simulink model "decisionTask"  (R2012b)
settings: Solver=FixedStepDiscrete  StartTime=0.0  StopTime=10.0  FixedStep=0.001  RelTol=1e-3
undefined symbols (not defined in the file or in its folder): acquireMethods, autoplayMovementDuration, autoplayReactionTime, autoplayRotationDuration, autoplayRotationStart, centerOffset, clickPercentage, clickRefractoryPeriod, clickTargetColor, clickTargetHoverColor, coherences, crossSize, cuedText, cuedTextLength, cumulativeDwell, cursorColorClick, cursorColorClosed, cursorColorOpen, cursorColors, cursorDiameter, cursorNeuralColor, cursorNonneuralColor, delayOrder, delayPeriodGainScale, displayObject, doHeadSpeedFail, drawNumbersOnTargets, dwellRefractoryPeriod, errorAssistAxis, errorAssistR, errorAssistTheta, expRandBinSize, expRandMax, expRandMin, expRandMu, eyeMode, failOnLiftoff, failurePenalty, falseClickFails, fingerPositionTolerance, fixedSeqMode, freePlayMode, gain, gloveBias, gloveLPDenominator, gloveLPNumerator, gloveNonlinearCorrection, gloveXCorrection, gloveYCorrection, gracePeriod, gridEdges, gridSize, gridTilesEachDim, headSpeedCap, holdDuration, holdTime, initialInput, initialLockout, initialState, inputType ... (+118)
(part 2 of 2)

== matlab function decisionTask/decisionTaskSplit ==
  data: xkRaw input double size=[double(xkConstants.NUM_STATE_DIMENSIONS) 1]; xkMod input; behaviorPacket input Bus: behaviorPacketBus size=1; vizData input Bus: peripheralData; taskOutput output Bus: taskOutput; stateParameters input Bus: stateParams size=1; decisionParameters input Bus: taskParamsBus; clock input; xpcTET input; xkModBiasEst input; taskAgnosticXk input; xkAux input
function taskOutput  = decisionTaskSplit(xkRaw, xkMod, behaviorPacket, vizData,  ...
    stateParameters, decisionParameters, clock, xpcTET, xkModBiasEst, taskAgnosticXk, xkAux)
% removed from input: clickState, clickParameters,
% should I change the connectors in the model to match this change? - SNF
%#codegen
% This is the state-machine-like implementation of the cursor task.
% This, depending on paraemters, can do center-out-and-back
%
% October 31 2016: now has two state inputs, xkRaw (which gets fed back to
% the decoder), and xkMod. Generally should look at xkMod for task logic,
% but if the game needs to change a state element which ought to propogate
% into the decoder (for example re-seed the cursor), it should do this to
% both xkRaw and xkMod.

% decisionParameters is actually taskParamsBus, which is set by
% cursotTask_buildWorkspace.m

%% INITIALIZE TASK OUTPUT - SNF to SNF: don't fuck with this.
fileLoggerData.data = uint8(zeros(1,1400));
fileLoggerData.dataLen = uint16(0);
fileLoggerData.fileName = uint8(zeros(1,20));
fileLoggerData.send = false;

fileLoggerFormat.format = uint8(zeros(1,1400));
fileLoggerFormat.formatLen = uint16(0);
fileLoggerFormat.fileName = uint8(zeros(1,20));

fileLoggerFormatAndData.format = fileLoggerFormat;
fileLoggerFormatAndData.data = fileLoggerData;

%% whether or not to allow the cursor to be stopped (e.g. during click)
% allowStop = true;
% resetHMM = false;

taskOutput.flushFiles = false;
taskOutput.sendFormat = false;
taskOutput.taskDetails = fileLoggerFormat;
taskOutput.discrete = fileLoggerFormatAndData;
taskOutput.continuous = fileLoggerFormatAndData;
taskOutput.screen = fileLoggerFormatAndData;
taskOutput.sound = fileLoggerFormatAndData;
taskOutput.asynch = fileLoggerFormatAndData;
taskOutput.ttl = double(0);
taskOutput.xk = xkRaw;
taskOutput.inputType = decisionParameters.initialInput;
taskOutput.currentTarget = single(zeros([double(xkConstants.NUM_TARGET_DIMENSIONS) 1]));
taskOutput.state = uint16(CursorStates.STATE_INIT);
taskOutput.paused = false;
taskOutput.allowStop =  true; %allowStop;
taskOutput.resetHMM = false; %resetHMM;

%% TASK DETAILS PACKET: SNF done for DM, builds successfully
TASK_NAME = 'decision';
VERSION_ID = single(0.01); % Alpha - SF

taskOutput.taskDetails = packFileLoggerTaskDetails(TASK_NAME, VERSION_ID, ...
    'STATE_INIT', uint8(CursorStates.STATE_INIT), ...
    'STATE_PRE_TRIAL', uint8(CursorStates.STATE_PRE_TRIAL),...
    'STATE_NEW_TARGET', uint8(CursorStates.STATE_NEW_TARGET),...
    'STATE_MOVE', uint8(CursorStates.STATE_MOVE),...
    'STATE_ACQUIRE', uint8(CursorStates.STATE_ACQUIRE),...
    'STATE_SUCCESS', uint8(CursorStates.STATE_SUCCESS),...
    'STATE_FAIL', uint8(CursorStates.STATE_FAIL),...
    'STATE_CENTER_TARGET', uint8(CursorStates.STATE_CENTER_TARGET),...
    'STATE_END', uint8(CursorStates.STATE_END),...
    'STATE_RECENTER_DELAY', uint8(CursorStates.STATE_RECENTER_DELAY),...
    'STATE_FIXATE', uint8(CursorStates.STATE_FIXATE),... %SNF DM state
    'STATE_STIMULUS_ONSET', uint8(CursorStates.STATE_STIMULUS_ONSET),... %SNF DM state
    'STATE_INTERTRIAL',  uint8(CursorStates.STATE_INTERTRIAL),... %SNF DM state
    'INPUT_TYPE_HEAD_MOUSE', uint8(cursorConstants.INPUT_TYPE_HEAD_MOUSE),...
    'INPUT_TYPE_CURSOR_HEADSTILL', uint8(cursorConstants.INPUT_TYPE_CURSOR_HEADSTILL),...%SF changed this 4/12
    'INPUT_TYPE_NONE', uint8(cursorConstants.INPUT_TYPE_NONE),... %SF: probably need this?
    'OUTPUT_TYPE_CURSOR', uint8(cursorConstants.OUTPUT_TYPE_CURSOR)...
    );

%% TASK-RELATED CONSTANTS
NUM_DIMS =  uint8(cursorConstants.NUM_DIMENSIONS); %this is 5
headCursorPos = single( zeros(1,NUM_DIMS) ); % head position cursor
cursorAlpha2 = uint8(100); % set to 100 if you're not using it. This is in %.

INIT_LENGTH = uint16(100); %ms
% PRE_TRIAL_LENGTH = uint16(20); %ms
SCORE_LENGTH = uint16(4000); %ms
INIT_TIME = uint32(2000); %this one's used explicitly for keeping pauseTriggered
MAX_MOVE_TIME = uint32(10000);
% HEAD_CURSOR_COLOR = [0; 204; 102;];
% AUTOPLAY_COLOR = [255; 255; 255];
EYE_X_SCALAR = 1680;
EYE_Y_SCALAR = 1050;
%HEAD_SCALAR = 1080; %this is only for offline I think
%%% DM specific
GRID_SIZE = 15*15; 
ISOGREEN = [0 90 0];
ISORED   = [160 0 0];
COLORMAT = [ISORED; ISOGREEN];
% trialConds: always L/D and Red first. 
% idx 1: 2 = L/R, 1 = U/D
% idx 2: color of left or down targ (depending on col 1) 2 = red, 3 = green
% idx 3: color of right or up targ  (depending on col 1) 2 = red, 3 = green
% idx 4: number of red squares (out of 225)
% idx 5: which target is correct. 1 = left/up, 2 = right/down
%indices into stimulus conditions matrix:
TARG_AXIS_IDX = 1;
LEFT_DN_TARG_COLOR_IDX = 2; %subtract 1 to get index for target order. left/down always first
RIGHT_UP_TARG_COLOR_IDX = 3; %always the second entry
NUM_RED_SQ_IDX = 4;
TARGET_LOC_IDX = 5;
% specifies what the values for each column mean:
LEFT_RIGHT_AXIS_TARGS = 2;
UP_DOWN_AXIS_TARGS = 1;
TARGET_RED = 2; %minus 1 to get row in COLORMAT
TARGET_GREEN = 3;  %minus 1 to get row in COLORMAT
LEFT_DN_TARG_S = 1;
RIGHT_UP_TARG_S = 2;
LEFT_DN_TARG_IDX = 1;
RIGHT_UP_TARG_IDX = 2;
% indices for activeTargs mask: could be more clever 
% DOWN_IDX = 1; why use these when the targAxis works
% LEFT_IDX = 2; 
% UP_IDX = 3; 
% RIGHT_IDX = 4;
CENTER_IDX = 5; 
% colors for those: 
TARGET_WHITE = 1;
TARGET_BLACK = 0; 
MIN_STIM_TIME = 300; 
%% DEFINE PERSISTENTS
persistent state vizPacket;
persistent pauseTriggered;
persistent stateTimer;
persistent holdTimer;
%persistent cursorColors; %this is defined in the task now
persistent targetRadiusTrans % added SDS Feb 2017, this is the target radius in XYZ
persistent targetRadiusRot % added SDS Feb 2017, this is the target radius in rotation
persistent currentTarget;
persistent nextTarget;
persistent speedCode;
persistent wiaCode; %this needs to stay for reasons SNF doesn't know

%persistent currentTargetType nextTargetType;  % dwell or click
persistent trialNum %cycleNum cycleIndex;
persistent trialDelayLength;

persistent localAcquired localTotal localTotalTime localAcqTime;
%persistent localScore totalScore;
persistent acquireTime lastState;

persistent lockedParameters inputType outputType;

persistent lastSoundTime;
persistent lastSoundState;

%persistent initialeffectorCursorPos; % previousInput;

persistent totalTaskTime;
%persistent lastAcquireSuccess 
persistent previousTarget;
persistent filteredHeadSpeed;
persistent prevHeadPos;
persistent lastHeadSpeedFail;

 
%DM-specific:
% persistent gracePeriod; % this should go in the params file SNF TO SDS HELP PLZ
% persistent maxStimDur; % ditto. 
persistent stimConds; % This didn't make it into the param script
% persistent moveThresh; % ditto again. 
% persistent intertrialTime; %last one- in the params plz
persistent trialConds;
persistent fixDur;  % variable timed
persistent targDur; % variable timed
persistent stimulusCount; %trialNum might replace this? 
persistent successPoints;
%defining targets:
persistent targAxis;
persistent targColors; %numTargs x RGB 
persistent targLocs;   %numTargs x XY
persistent autoTarg; % 1 or 2 for L/D or R/U 
%defining stimulus:
persistent numRedSquares; 
persistent activeTargs; 
persistent maxFixateAttemptTime; 
persistent fixateAttemptTimer; 
persistent autoCursorPos; 
%% grab these off the bus: 

behaviorRequestClock = behaviorPacket.xpcRequestClock;
peripheralTimestamp = behaviorPacket.peripheralTimestamp(1:16);

%% INITIALIZE PERSISTENTS
if(isempty(state))
    state = uint16(CursorStates.STATE_INIT);
    lastState = state;
    currentTarget = single(zeros([double(xkConstants.NUM_TARGET_DIMENSIONS) 1]));
    nextTarget = single(zeros([double(xkConstants.NUM_TARGET_DIMENSIONS) 1]));
    
    speedCode = uint16(0); %FRW hacky instructed speed experiment
    wiaCode = uint16(0); %FRW hacky wia experiment
    vizPacket = initVizPacket;
    stateTimer = uint16(0);
    holdTimer = int16(0);
    pauseTriggered = true;
    
  %  cursorColors = double(zeros([3 3])); % there's a second cursor (column 2) allowed; now a third for eye cursor
    filteredHeadSpeed = single(0);
    prevHeadPos = single(zeros(2,1));
    
    %% buffer all the parameters off the bus
    lockedParameters = decisionParameters;
    stimConds = getStimMat(double(lockedParameters.coherences)); %this only happens once per run of the task.
    targetRadiusTrans = (double(lockedParameters.targetDiameter) / 2) +(double(lockedParameters.cursorDiameter) / 2);
    targetRadiusRot = double(lockedParameters.targetRotDiameter) / 2;
    
    inputType = lockedParameters.initialInput;
    trialNum = uint16(0);
  %  cycleNum = uint16(0);
  %  cycleIndex = uint16(1); % 1 so it's a valid idnex even when first used
    trialDelayLength = uint16(0);
    
    localTotal = uint16(0);
    localTotalTime = uint16(0);
    localAcquired = uint16(0);
    localAcqTime = uint16(0);
    acquireTime = stateTimer;
   % currentTargetType = uint16(cursorConstants.TARGET_TYPE_DWELL);
    nextTargetType = uint16(cursorConstants.TARGET_TYPE_DWELL);
    %SFstateBeforePreTrial = uint16(0);
    lastSoundTime = clock;
    lastSoundState = uint8(CursorStates.SOUND_STATE_IDLE);

    
    totalTaskTime = uint32(0);
    lastHeadSpeedFail = uint32(0);
    
 %   lastAcquireSuccess = false;
    previousTarget = currentTarget;
    % DM-specific: 
    fixDur = uint16(0); 
    targDur = uint16(0); 
    successPoints = uint16(0);
    stimulusCount = uint16(1); 
    %initialize stimulus conditions
    targAxis = uint16(LEFT_RIGHT_AXIS_TARGS);
    trialConds = uint16(zeros(1,5));
    targColors = uint16(zeros(2, 3)); 
    targColors(LEFT_DN_TARG_COLOR_IDX -1,:)  = uint16(ISORED); % if I see two red targets I know it's a problem
    targColors(RIGHT_UP_TARG_COLOR_IDX -1,:) = uint16(ISORED); % but we at least got here
    numRedSquares = uint16(GRID_SIZE); %if all red, again, we know we got here. 
    targLocs = single(zeros(2,2)); 
    targLocs(:, LEFT_DN_TARG_COLOR_IDX -1) = single([-1; -1]); %one target in the lower left, one in upper right. Col = targ
    targLocs(:, RIGHT_UP_TARG_COLOR_IDX -1) = single([1; 1]);
   % gracePeriod = uint16(200); %ms
    autoTarg = uint16(0); % no target
   % maxStimDur = uint16(0); 
   % moveThresh = uint16(200); %units of idk mate
   % intertrialTime = uint16(1000); %ms 
 %  activeTargs = logical(false(1,5)); 
   activeTargs = uint16(zeros(1,5)); 
   maxFixateAttemptTime = uint16(5000); %ms
   fixateAttemptTimer = uint16(0); 
   autoCursorPos =  double(zeros(5,1));
end

%% some more initialization
if(clock < INIT_TIME) %1 whole second
    pauseTriggered = true;
end
%% inits per loop: 
outputType = decisionParameters.outputType; % determines what graphics engine will render this task.
% We usually shouldn't write discrete data
writeDiscreteData = false; %only gets set to true in state_pre_trial once
writeContinuousData = true;

if(vizData.receive && (vizData.dataLen > 0 ))
    vizPacket = parseVizPacket(vizData.data);
end

% set the cursor and target color
% if uint16(inputType) == uint16(cursorConstants.INPUT_TYPE_HEAD_MOUSE)
%     cursorColors(1:end,1) = [0; 204; 102;]; %head position is always green
% elseif  uint16(inputType) == uint16(cursorConstants.INPUT_TYPE_AUTO_ACQUIRE)
%     cursorColors(1:end,1) = [255; 255; 255]; % BCI control
% end
targetColor = 'a'; % in other tasks, target still aqua
makeGridFlag = uint16(0);
% init target logic- transient 
translateOnTargetLD = false; 
translateOnTargetRU = false; 
%% some end effector maths
% which state elements do I look to for the cursor's position? SDS July 2016
xk2HorizontalPos = uint8( lockedParameters.xk2HorizontalPos );
xk2VerticalPos = uint8( lockedParameters.xk2VerticalPos );
xk2HorizontalVel = uint8( lockedParameters.xk2HorizontalVel );
xk2VerticalVel = uint8( lockedParameters.xk2VerticalVel );
xk2DepthPos = uint8( lockedParameters.xk2DepthPos );
xk2DepthVel = uint8( lockedParameters.xk2DepthVel );
xk2RotatePos = uint8( lockedParameters.xk2RotatePos );
xk2RotateVel = uint8( lockedParameters.xk2RotateVel );
xk2Rotate2Pos = uint8( lockedParameters.xk2Rotate2Pos );
xk2Rotate2Vel = uint8( lockedParameters.xk2Rotate2Vel );
TASK_DIMS = lockedParameters.numDisplayDims; % 2. only used for determining what kind of
% checking to use. We still need to have everything be NUM_DIMS (5) long or
% things won't compile.
canBePosInds = [xk2HorizontalPos,xk2VerticalPos,xk2DepthPos,xk2RotatePos,xk2Rotate2Pos];
canBeVelInds = [xk2HorizontalVel,xk2VerticalVel,xk2DepthVel,xk2RotateVel,xk2Rotate2Vel];
effectorPosInds = canBePosInds(1:NUM_DIMS);
effectorVelInds = canBeVelInds(1:NUM_DIMS);

%displayAuxCursor = false;
if uint16(inputType) == uint16(cursorConstants.INPUT_TYPE_HEAD_MOUSE)
    effectorPos = xkMod(effectorPosInds); %Head position is the main effector
    effectorVel = xkMod(effectorVelInds); %lol head vel not saved
    %auxEffectorPos = xkMod(effectorPosInds); %BCI is auxilary. 
    %auxEffectorPos = zeros(NUM_DIMS,1);    %Actually no, we don't care about BCI
    auxEffectorPos = effectorPos; %make this easy for SNF and PTB- always send head pos as cursor2
    %displayAuxCursor = true; %the head cursor *is* the cursor, so no aux
    %cursorColors(:,2) = AUTOPLAY_COLOR; %HEAD_CURSOR_COLOR; %SF doesn't want a green cursor in a red/green task
%elseif uint16(inputType) == uint16(cursorConstants.INPUT_TYPE_AUTO_ACQUIRE)
elseif uint16(inputType) == uint16(cursorConstants.INPUT_TYPE_CURSOR_HEADSTILL)
    effectorPos = xkMod(effectorPosInds); %BCI is the main effector
    effectorVel = xkMod(effectorVelInds);
    auxEffectorPos = xkAux(effectorPosInds); %head mouse is auxEffector
    %displayAuxCursor = true; %only show head cursor during fixation
    %cursorColors(:,2) = AUTOPLAY_COLOR; % BCI control
else %default to BCI and dgaf about head position
    effectorPos = xkMod(effectorPosInds);
    effectorVel = xkMod(effectorVelInds);
    auxEffectorPos = zeros(NUM_DIMS,1);
end

%% head speed check
% we low pass filter the 1ms head speed and can fail the trial if it is too high
headSpeedAlpha = single(0.96);
headSpeed = 1000*sqrt(sum((behaviorPacket.windowsMousePosition - prevHeadPos).^2));
filteredHeadSpeed = headSpeedAlpha*filteredHeadSpeed + (1-headSpeedAlpha)*headSpeed;
prevHeadPos = behaviorPacket.windowsMousePosition;

%SF: this is copied into the relevant parts of the state machine
%play fail sound if moving the head when he shouldn't be
% if lockedParameters.doHeadSpeedFail && (filteredHeadSpeed > lockedParameters.headSpeedCap) ...
%         &&((clock - lastHeadSpeedFail)>2000)
%     %stateTimer = uint16(0);
%     %state = uint16(CursorStates.STATE_FAIL);
%     lastHeadSpeedFail = clock;
%     lastSoundTime = clock;
%     lastSoundState = uint8(CursorStates.SOUND_STATE_FAIL);
% end
%% get the eye position so it can get saved (as eyeCursorPos)
eyePos = behaviorPacket.windowsPC1GazePoint;
eyePos(1) = (eyePos(1)-0.5)*EYE_X_SCALAR;
eyePos(2) = (eyePos(2)-0.5)*EYE_Y_SCALAR;

eyeCursorPos = single(nan(NUM_DIMS,1)); %need this for output -SNF
eyeCursorPos(1:2) = eyePos; %[eyePos(1), eyePos(2)];
%%
%--the auxiliary cursor must be in the center to acquire a target with the
%actual cursor
%--in modes where the aux. cursor is not used, its position is zero, placing
%it in the center so it will pass all auxInCenter checks
% auxInCenter = sqrt(sum(auxEffectorPos.^2))<80; %Frank, no magic numbers

%display auxiliary cursor
%if displayAuxCursor
%     headCursorPos = single(auxEffectorPos);
%end

%% generally, allow cursor to stop off target. check options
% allowStop = lockedParameters.stopOffTarget;

%SF if clock> INIT_TIME && state~= uint16(CursorStates.STATE_INIT) && state ~= uint16(CursorStates.STATE_CENTER_TARGET)
%     % Game is locked awaiting finger liftoff. Old stuff that Chethan/Paul
%     % wrote, I don't know what it really does or why. -Sergey
%SF  %SF   previousInput = inputType;
%     state = uint16(CursorStates.STATE_FINGER_MOVED);
%     cursorColors(1:end,1) = [255;133;0];
%     stateTimer = uint16(0);
%     currentTarget(1:NUM_DIMS,:) = single(initialeffectorCursorPos);
%SF else
%SF:
%if clock >= INIT_TIME % this maintains the if/else-ness from the above sh
%%%%%%% STATE MACHINE
switch state
%% INITIALIZE BLOCK:
    case {CursorStates.STATE_INIT}
        %enter this state at the start of each **BLOCK**
        % set all the persistents that may have been changed by user input
        pauseTriggered = stateParameters.pause; %SF deems pause not worth cutting
        lockedParameters = decisionParameters;
        writeContinuousData = false;
        inputType = lockedParameters.initialInput;
        % generate some entropy
        jnk = rand(1,1);
      %  initialCursorPos = single( zeros(NUM_DIMS,1) );
        if ~pauseTriggered
            stateTimer = stateTimer + 1;
        else
            jnk = rand(1,1); %more entropy depending on how long it's paused
        end
        
        if stateTimer >= INIT_LENGTH %100 ms
            stateTimer = uint16(0);
            trialNum = uint16(0);
            currentTarget(:) = single(zeros(double(xkConstants.NUM_TARGET_DIMENSIONS),1));
          %  cycleNum = uint16(0); %number of iterations within a block?
            %start SF state code:
            %get stimConds from lockedParams: %SF edit: initialized earlier
            % stimConds = lockedParameters.stimulusMat;
            state = uint16(CursorStates.STATE_PRE_TRIAL);
        end
%% GET TRIAL INFO:
    case {CursorStates.STATE_PRE_TRIAL} %runs once per trial for 100 ms
        if stateTimer == 0
            pauseTriggered = stateParameters.pause;
            %stateBeforePreTrial = lastState;
        end
        if ~pauseTriggered %ugh @ pauseTriggered
            stateTimer = stateTimer + 1;
        end
        % reset the stim counter if we've finished a block
        if stimulusCount > lockedParameters.numTrials % trialNum > lockedParameters.numTrials %if this block is over
            stimulusCount = uint16(1);
            stimConds = getStimMat(double(lockedParameters.coherences));
        end
        if stateTimer == 1 % for things that happen once per trial
            lockedParameters = decisionParameters;
            targetRadiusTrans = (double(lockedParameters.targetDiameter) / 2) + (double(lockedParameters.cursorDiameter)/2);
            targetRadiusRot = double(lockedParameters.targetRotDiameter) / 2;
            writeDiscreteData = true; %do this once per trial
            makeGridFlag =  uint16(1);  
            % get **trial's** entry from stimConds
            trialConds = uint16(stimConds(stimulusCount,:)); %get the trial's stim and targ values
        %get target locations
            targAxis = uint16(trialConds(TARG_AXIS_IDX)); %are they going to be up/downs (1) or left/rights (2)?
            %targLocs = lockedParameters.targetInds(1:2, targAxis:2:end);
            %splitting this ^^ up for readability:
            targLocs(:, LEFT_DN_TARG_COLOR_IDX -1)  = lockedParameters.targetInds(1:2, targAxis); %1 or 2
            targLocs(:, RIGHT_UP_TARG_COLOR_IDX -1) = lockedParameters.targetInds(1:2, targAxis+2); %3 or 4
            %get RGB colors for targets:
            targColors(LEFT_DN_TARG_COLOR_IDX -1, :) = COLORMAT(uint16(trialConds(LEFT_DN_TARG_COLOR_IDX))-1,:)'; %get target colors
            targColors(RIGHT_UP_TARG_COLOR_IDX -1,:) = COLORMAT(uint16(trialConds(RIGHT_UP_TARG_COLOR_IDX))-1,:)';
            %GET THIS ^^^ TO PBT but don't display it yet
        end
        
        if stateTimer >= lockedParameters.preTrialLength %if we've exhausted this state
            stateTimer = uint16(0);
            %SF: trailNum increments at the STIM state

            %set the variable  delay for fixation
            if lockedParameters.useRandomDelay
                % pick a new random delay
                while double(trialDelayLength) < lockedParameters.expRandMin || double(trialDelayLength) > lockedParameters.maxFixDur
                    trialDelayLength = uint16(lockedParameters.expRandMu * -log(rand([1 1])));
                end
                trialDelayLength = uint16(round(double(trialDelayLength) / double(lockedParameters.expRandBinSize))*lockedParameters.expRandBinSize);
            else
                trialDelayLength = uint16(lockedParameters.expRandMu);
            end
            fixDur = trialDelayLength;
            trialDelayLength = uint16(0); %reset to 0 now that fixDur is set
            state = uint16(CursorStates.STATE_FIXATE); %on to the actual task
        end
        

%% CENTER HEAD AND FIXATE:
    case CursorStates.STATE_FIXATE
        % hold here until the head and eyes are centered, showing head pos
        % start a variable delay timer once head is centered and still
        %currentTarget = centerHold; %SNF: look up centerHold values. I hope it's [0, 0].
        % SNF: centerHold doesn't exist...
        currentTarget = single(zeros([double(xkConstants.NUM_TARGET_DIMENSIONS) 1])); %fixate at [0,0]
      %  displayAuxCursor = true; %this is unused so.... do this instead: 
        cursorAlpha2 = uint8(0); %set cursor 2 to visible 
        %SNF: this logic here... does this mean if he makes minor corrections
        % immediately after entering the target he'll fail?
        % SNF replies: added gracePeriod to get around this (ungracefully)
       % activeTargs(CENTER_IDX) = uint16(TARGET_WHITE); %switched to fixation cross
        activeTargs(CENTER_IDX) = uint16(TARGET_BLACK);  %but does he still need a target? 
        % if he's on the target, start a timer to hold and fail if he moves too much
        if isCursorOnTarget(prevHeadPos, double(lockedParameters.cursorDiameter)/2, currentTarget, targetRadiusTrans, TASK_DIMS)
            %fail if moving the head when he should be holding
               %lastSoundTime = clock;
                %lastSoundState = uint8(CursorStates.SOUND_STATE_GO);
            if (stateTimer > lockedParameters.gracePeriod) && (lockedParameters.doHeadSpeedFail) && (filteredHeadSpeed > lockedParameters.headSpeedCap) ...
                    &&  ((clock - lastHeadSpeedFail)>2000)
                %go to fail state
                stateTimer = uint16(0);
                state = uint16(CursorStates.STATE_FAIL);
                fixDur = uint16(0); %reset for the next trial
                % reset fail clocks
                lastHeadSpeedFail = clock;
                %lastSoundTime = clock;
                %lastSoundState = uint8(CursorStates.SOUND_STATE_FAIL);
            elseif stateTimer < fixDur %holding still for random delay
                stateTimer = stateTimer + 1;
            else % if we've exhausted the fix time, present targets or stimulus!
                fixDur = uint16(0); %reset this
                if lockedParameters.taskOrder == uint16(decisionConstants.TASK_TARG_FIRST)
                    state = uint16(CursorStates.STATE_NEW_TARGET); %Formerly known as TARGETS_ONSET
                else
                    state = uint16(CursorStates.STATE_STIMULUS_ONSET);
                    activeTargs = uint16(zeros(1,5)); %make sure no targets appear yet
                end
                    stateTimer = uint16(0);
                %set the variable  delay for targets 
                %(or delay period if stimulus first, -SF 06/18)
                if ~trialDelayLength %&& ~all(nextTarget==0)
                    if lockedParameters.useRandomDelay
                        % pick a new random delay
                        while double(trialDelayLength) < lockedParameters.expRandMin || double(trialDelayLength) > lockedParameters.maxTargDur
                            trialDelayLength = uint16(lockedParameters.expRandMu * -log(rand([1 1])));
                        end
                        trialDelayLength = uint16(round(double(trialDelayLength) / double(lockedParameters.expRandBinSize))*lockedParameters.expRandBinSize);
                        %targDur = trialDelayLength;
                    else
                        trialDelayLength = uint16(lockedParameters.expRandMu);
                    end
                end
                targDur = trialDelayLength;
                trialDelayLength = uint16(0); %reset to 0 now that targDur is set
            end
        else % stay in this state indefinitely until he gets his head to the center target
            %this else clause is probs uneccessary
            fixateAttemptTimer = uint16(fixateAttemptTimer + 1); 
            if fixateAttemptTimer > maxFixateAttemptTime
                state = uint16(CursorStates.STATE_FAIL); 
                fixateAttemptTimer = uint16(0); 
            else
                state = uint16(CursorStates.STATE_FIXATE);
            end
        end
        
%% SHOW TARGETS: AKA TARGETS_ONSET
    case {CursorStates.STATE_NEW_TARGET}
        %stateTimer = stateTimer + 1;
        %fail if moving the head when he shouldn't be
        % set the visibility of the targets to be displayed to be on:
        activeTargs(targAxis) = uint16(trialConds(LEFT_DN_TARG_COLOR_IDX)); %entry from trialConds that specifies targ1 color
        activeTargs(targAxis + 2) = uint16(trialConds(RIGHT_UP_TARG_COLOR_IDX)); %entry from trialConds that specifies targ2 color
        %         if stateTimer == 1
        %             auxEffectorPos = zeros(1,5);
        %             effectorPos = zeros(1,5);
        %         end
        if lockedParameters.taskOrder == uint16(decisionConstants.TASK_TARG_FIRST) %normal case: 
            % hold still while targets are on
            if (lockedParameters.doHeadSpeedFail) && (filteredHeadSpeed > lockedParameters.headSpeedCap) ...
                    &&  ((clock - lastHeadSpeedFail)>2000)
                %go to fail state
                stateTimer = uint16(0);
                targDur = uint16(0);
                state = uint16(CursorStates.STATE_FAIL);
                % reset fail clocks
                lastHeadSpeedFail = clock;
                % lastSoundTime = clock;
                % lastSoundState = uint8(CursorStates.SOUND_STATE_FAIL);
            elseif stateTimer < targDur %loop while holding still
                stateTimer = stateTimer + 1;
            else %if we've timed this state out without moving, onward!
                xkMod([effectorPosInds, effectorVelInds],1) = 0;
                xkRaw([effectorPosInds, effectorVelInds],1) = 0; %sure hope this is enough
                state = uint16(CursorStates.STATE_STIMULUS_ONSET);
                stateTimer = uint16(0);
                targDur = uint16(0);
            end
        else % if stimulus first, target onset is cue to move
            stateTimer = stateTimer + 1;
           switch lockedParameters.taskType
                case uint32(cursorConstants.TASK_BCI_REPORT)
                    % If BCI: start decoding vel
                    % if BCI, enforce head still
                    if (lockedParameters.doHeadSpeedFail) && (filteredHeadSpeed > lockedParameters.headSpeedCap) ...
                            &&  ((clock - lastHeadSpeedFail)>2000)
                        %go to fail state
                        stateTimer = uint16(0);
                        state = uint16(CursorStates.STATE_FAIL);
                        % reset fail clocks
                        lastHeadSpeedFail = clock;
                    % if the checkerboard has been up long enough and we decode movement, go to move state    
                    elseif(stateTimer > MIN_STIM_TIME) && (sqrt(effectorVel(1)^2 + effectorVel(2)^2) > (lockedParameters.moveThresh)) %(lockedParameters.moveThresh/10000)) %lockedParameters.moveThresh % move to targ if a big vel is sent
                        xkMod([effectorPosInds, effectorVelInds],1) = 0;
                        xkRaw([effectorPosInds, effectorVelInds],1) = 0;
                        stimulusCount = stimulusCount + 1;
                        state = uint16(CursorStates.STATE_MOVE);
                        stateTimer = uint16(0);
                    % "max stim dur" is max deliberation time, basically,
                    % so it's an appropriate length here, even though it's
                    % poor naming convention form: 
                    elseif stateTimer > lockedParameters.maxStimDur
                        % if timeout, fail in BCI case
                        state = uint16(CursorStates.STATE_FAIL);
                        stateTimer = uint16(0);
                        %if we saw the stimulus, skip it?
                        stimulusCount = stimulusCount + 1;
                    end
                    
                case uint32(cursorConstants.TASK_HEAD_REPORT)
                    % if you move erroneously soon
                    if (stateTimer < MIN_STIM_TIME) && headSpeed > lockedParameters.headSpeedCap %if we exceed the threshold we declared for failing
                        state = uint16(CursorStates.STATE_FAIL);
                        stateTimer = uint16(0);
                        %if not erroneously soon:
                    elseif headSpeed > lockedParameters.headSpeedCap %if we exceed the threshold we declared for failing
                        state = uint16(CursorStates.STATE_MOVE);
                        stimulusCount = stimulusCount + 1;
                        stateTimer = uint16(0);
                    elseif stateTimer > lockedParameters.maxStimDur %force decision when undecided in head control
                        % effectorPos = zeros(1,5); %keep BCI position centered to start the next movement
                        state = uint16(CursorStates.STATE_MOVE);
                        stimulusCount = stimulusCount + 1;
                        stateTimer = uint16(0);
                        
                    end
            end
        end
%% SHOW THE COLOR GRID 
    case CursorStates.STATE_STIMULUS_ONSET
        % extinguish fixation, draw grid in PTB
        numRedSquares = uint16(trialConds(NUM_RED_SQ_IDX));
        %start monitoring BCI or head vel
        % if movement effector > thresh, enter TARGET_ACQUIRE
        stateTimer = stateTimer + 1;
        activeTargs(CENTER_IDX) = uint16(TARGET_BLACK); %make center target disappear
        
        if lockedParameters.taskOrder == uint16(decisionConstants.TASK_TARG_FIRST)
            % effectorPos = zeros(1,5)'; %keep BCI cursor position centered here
            switch lockedParameters.taskType
                case uint32(cursorConstants.TASK_BCI_REPORT)
                    % effectorVel = xkMod(effectorVelInds);
                    % If BCI: start decoding vel
                    % if BCI, enforce head still
                    if (lockedParameters.doHeadSpeedFail) && (filteredHeadSpeed > lockedParameters.headSpeedCap) ...
                            &&  ((clock - lastHeadSpeedFail)>2000)
                        %go to fail state
                        stateTimer = uint16(0);
                        state = uint16(CursorStates.STATE_FAIL);
                        % reset fail clocks
                        lastHeadSpeedFail = clock;
                        
                    elseif(stateTimer > MIN_STIM_TIME) && (sqrt(effectorVel(1)^2 + effectorVel(2)^2) > (lockedParameters.moveThresh)) %(lockedParameters.moveThresh/10000)) %lockedParameters.moveThresh % move to targ if a big vel is sent
                        xkMod([effectorPosInds, effectorVelInds],1) = 0;
                        xkRaw([effectorPosInds, effectorVelInds],1) = 0;
                        stimulusCount = stimulusCount + 1;
                        state = uint16(CursorStates.STATE_MOVE);
                        stateTimer = uint16(0);
                    elseif stateTimer > lockedParameters.maxStimDur
                        % if timeout, fail in BCI case
                        state = uint16(CursorStates.STATE_FAIL);
                        stateTimer = uint16(0);
                        %if we saw the stimulus, skip it?
                        stimulusCount = stimulusCount + 1;
                    end
                    
                case uint32(cursorConstants.TASK_HEAD_REPORT)
                    % if you move erroneously soon
                    if (stateTimer < MIN_STIM_TIME) && headSpeed > lockedParameters.headSpeedCap %if we exceed the threshold we declared for failing
                        state = uint16(CursorStates.STATE_FAIL);
                        stateTimer = uint16(0);
                        %if not erroneously soon:
                    elseif headSpeed > lockedParameters.headSpeedCap %if we exceed the threshold we declared for failing
                        state = uint16(CursorStates.STATE_MOVE);
                        stimulusCount = stimulusCount + 1;
                        stateTimer = uint16(0);
                    elseif stateTimer > lockedParameters.maxStimDur %force decision when undecided in head control
                        % effectorPos = zeros(1,5); %keep BCI position centered to start the next movement
                        state = uint16(CursorStates.STATE_MOVE);
                        stimulusCount = stimulusCount + 1;
                        stateTimer = uint16(0);
                        
                    end
            end
        else %if it's checkerboard first, always enforce head fixation and start a timer
            activeTargs = uint16(zeros(1,5)); %make really sure there are no targets
            if stateTimer > lockedParameters.stimDur
                state = uint16(CursorStates.STATE_DELAY); %variable delay before target onset
                stimulusCount = stimulusCount + 1;
                stateTimer = uint16(0);
            elseif (filteredHeadSpeed > lockedParameters.headSpeedCap) ...
                    &&  ((clock - lastHeadSpeedFail)>2000)
                %go to fail state
                stateTimer = uint16(0);
                state = uint16(CursorStates.STATE_FAIL);
                % reset fail clocks
                lastHeadSpeedFail = clock;
            else
                stateTimer = stateTimer + 1;
            end
            
        end
%% STATE_DELAY
case {CursorStates.STATE_DELAY}
    stateTimer = stateTimer + 1;
    %checkerboard needs to be blanked here, that's a problem for PTB
    if  (filteredHeadSpeed > lockedParameters.headSpeedCap) ...
            &&  ((clock - lastHeadSpeedFail)>2000)
        %go to fail state
        stateTimer = uint16(0);
        state = uint16(CursorStates.STATE_FAIL);
        % reset fail clocks
        lastHeadSpeedFail = clock;
    end
    if stateTimer > targDur
        stateTimer = uint16(0);
        state = uint16(CursorStates.STATE_NEW_TARGET);
    end
%% STATE_MOVE
    case {CursorStates.STATE_MOVE}
%hang out and wait for a cursor to get to the target
% move the cursor toward the target if BCI mode. 
        stateTimer = stateTimer + 1;
        % wait here until the cursor is over a target
        % if cursor over either target, judge target for success
        
        % we're doing autoplay ourselves here if BCI:
      % start the cursors in the center
        if stateTimer == 1
          xkMod([effectorPosInds, effectorVelInds],1) = 0;
          xkRaw([effectorPosInds, effectorVelInds],1) = 0;
        end
% % 
% %         % xkoutRaw(effectorTransPosInds) = xkStart(effectorTransPosInds) -  xTgt(1:NUM_TRANS_DIMS)* double( (15*tau^4 - 6*tau^5 - 10*tau^3) );
%          if lockedParameters.taskType == uint8(cursorConstants.TASK_BCI_REPORT) %lockedParameters.taskType == uint32(cursorConstants.TASK_BCI_REPORT)
%             autoCursorPos(1:2) = double(autoCursorPos(1:2)) + effectorVel(1:2);
%             effectorPos(1:2) = double(autoCursorPos(1:2)); 
%          end
             %             % zero unused dimension
%             if targAxis == UP_DOWN_AXIS_TARGS %if targs are up down, zero X
%                 potent = 2;
%                 null = 1;
%             else %if they're left-right, zero y (make it null)
%                 potent = 1;
%                 null = 2;
%             end
             % increment for the direction we're going
%             tau = lockedParameters.tau;
%             if autoTarg == RIGHT_UP_TARG_IDX
%                 autoCursorPos(potent) = autoCursorPos(potent) - targLocs(potent, RIGHT_UP_TARG_IDX)* double( (15*tau^4 - 6*tau^5 - 10*tau^3) );
%                 autoCursorPos(null) = 0;
%             else % if moving left:
%                 autoCursorPos(potent) = autoCursorPos(potent) - targLocs(potent, LEFT_DN_TARG_IDX)* double( (15*tau^4 - 6*tau^5 - 10*tau^3) );
%                 autoCursorPos(null) = 0;
%             end
%             % now reset the value of effectorPos bc I think it's getting
%             % overwritten with xkMod crap each iteration 
%             effectorPos = autoCursorPos; 
%         end
        
        % see if that step (or the head position) got us onto the target (edge of the cursor touched edge of target
        translateOnTargetLD = isCursorOnTarget(effectorPos, double(lockedParameters.cursorDiameter)/2,...
                                        targLocs(:,LEFT_DN_TARG_IDX), targetRadiusTrans, TASK_DIMS);
        translateOnTargetRU = isCursorOnTarget(effectorPos, double(lockedParameters.cursorDiameter)/2,...
                                        targLocs(:,RIGHT_UP_TARG_IDX), targetRadiusTrans, TASK_DIMS);
        
        if translateOnTargetLD || translateOnTargetRU
           % if lockedParameters.taskType == uint8(cursorConstants.TASK_HEAD_REPORT)
                 if targAxis == uint16(UP_DOWN_AXIS_TARGS)
                     decodeDirection = effectorPos(2); %taking the sign of Y pos at targ
                 else
                     decodeDirection = effectorPos(1); %taking the sign of X pos at targ
                 end
                 if decodeDirection < 0
                     autoTarg = uint16(LEFT_DN_TARG_IDX); % Left or down
                 else
                     autoTarg = uint16(RIGHT_UP_TARG_IDX); % right or up
                 end
           % end
            state = uint16(CursorStates.STATE_ACQUIRE); 
            stateTimer = uint16(0);
        %    autoCursorPos = zeros(5,1); 
        end
        if stateTimer > MAX_MOVE_TIME
            stateTimer = uint16(0); 
            state = uint16(CursorStates.STATE_FAIL); 
        %    autoCursorPos = zeros(5,1); 
        end
        
%% A TARGET WAS ACQUIRED - JUDGE IF IT WAS THE CORRECT ONE
    case {CursorStates.STATE_ACQUIRE}
         %judging - only takes one iteration
        stateTimer = stateTimer + 1; %therefore this is not needed
   
        if ( uint16(trialConds(TARGET_LOC_IDX)) == uint16(LEFT_DN_TARG_S)) && (autoTarg == LEFT_DN_TARG_IDX)% success for left or down and vel is left or down
            state =  uint16(CursorStates.STATE_SUCCESS);
            stateTimer = uint16(0); 
        elseif ( uint16(trialConds(TARGET_LOC_IDX)) == uint16(RIGHT_UP_TARG_S)) && (autoTarg == RIGHT_UP_TARG_IDX)% success for right or up and vel is right or up
            state =  uint16(CursorStates.STATE_SUCCESS);
            stateTimer = uint16(0); 
        else
            state = uint16(CursorStates.STATE_FAIL); 
            stateTimer = uint16(0); 
        end    
%% CENTER CURSORS- unused for now
    case {CursorStates.STATE_CENTER_TARGET}
       stateTimer = stateTimer + 1;
       currentTarget(:) = single(zeros(double(xkConstants.NUM_TARGET_DIMENSIONS),1));
        %    initialeffectorCursorPos = single( effectorPos ); % the (1:NUM_DIMS) is to handhold compilter about the dimensionality
           if isCursorOnTarget(effectorPos, double(lockedParameters.cursorDiameter)/2, currentTarget, targetRadiusTrans, TASK_DIMS)
                state = uint16(CursorStates.STATE_INTERTRIAL);
                stateTimer = uint16(0);
           end
           activeTargs = uint16(zeros(1,5)); 
%% STATE_RECENTER_DELAY- unused for now
    case {CursorStates.STATE_RECENTER_DELAY}
        stateTimer = stateTimer + 1;
        if stateTimer <= lockedParameters.recenterDelay
            xkMod(effectorPosInds,1) = previousTarget(1:NUM_DIMS);
            xkRaw(effectorPosInds,1) = previousTarget(1:NUM_DIMS);
            xkMod(effectorVelInds,1) = 0;
            xkRaw(effectorVelInds,1) = 0;
        else
            if lockedParameters.soundOnGo
                lastSoundTime = clock;
                lastSoundState = uint8(CursorStates.SOUND_STATE_GO);
            end
            stateTimer = uint16(0);
            state = uint16(CursorStates.STATE_INTERTRIAL);
        end
        activeTargs = uint16(zeros(1,5)); 

%% STATE_SUCCESS
    case {CursorStates.STATE_SUCCESS}
        stateTimer = stateTimer + 1;
        inputType = lockedParameters.inputType;
        trialNum = trialNum+1;
        successPoints = successPoints + 1; 
        % how do we score this trial?
        localAcquired = localAcquired + 1;
        localTotalTime = localTotalTime + acquireTime;
        
        localAcqTime = uint16(single(localTotalTime) / single(localTotal));
       % lastAcquireSuccess = true;
        
        if lockedParameters.soundOnSuccess && stateTimer <= 1
            lastSoundTime = clock;
            lastSoundState = uint8(CursorStates.SOUND_STATE_SUCCESS);
        end
        activeTargs = uint16(zeros(1,5));        
        stateTimer = uint16(0);
            state = uint16(CursorStates.STATE_INTERTRIAL);
        
%% STATE_FAIL
    case {CursorStates.STATE_FAIL}
        stateTimer = stateTimer + 1;
        inputType = lockedParameters.inputType;
        trialNum = trialNum+1;
       % lastAcquireSuccess = false;
        if lockedParameters.soundOnFail && stateTimer <= 1 % second condition is so failure sound played just once
            lastSoundTime = clock;
            lastSoundState = uint8(CursorStates.SOUND_STATE_FAIL);
        end
        activeTargs = uint16(zeros(1,5)); 
        stateTimer = uint16(0);
            state = uint16(CursorStates.STATE_INTERTRIAL);
        
%% ITI 
    case {CursorStates.STATE_INTERTRIAL}
        stateTimer = stateTimer + 1;
        if stateTimer >= lockedParameters.intertrialTime
            currentTarget(:) = single(zeros(double(xkConstants.NUM_TARGET_DIMENSIONS),1));
            
            state =  uint16(CursorStates.STATE_PRE_TRIAL);
            stateTimer = uint16(0); 
        end
        activeTargs = uint16(zeros(1,5)); 
%% STATE_END
    case {CursorStates.STATE_END}
        stateTimer = stateTimer + 1;
        %this hangs here foreverrrrrrrr 
        %make sure the cursors and targets disappear 
        % gracefully end the block? 
end
%%%%END STATE MACHINE
%%
% if the max block time reached, end the block: 
if lockedParameters.maxTaskTime && totalTaskTime > lockedParameters.maxTaskTime
    state = uint16(CursorStates.STATE_END);
end
if ~pauseTriggered
    totalTaskTime = totalTaskTime+1;
end
taskOutput.xk = xkRaw; % feed *raw* xk back out, which goes to decoder and file logger
taskOutput.currentTarget = single(currentTarget(:,1));
taskOutput.state = state;

% make sure we send the compiled dimension size, but only fill the used
% task ones.
effectorCursorPos = single(effectorPos'); %these are all 1 x 5
cursorVelocity = single(effectorVel');
taskAgnosticVel = single(taskAgnosticXk(effectorVelInds)'); 
headCursorPos = single(auxEffectorPos); %1 x 5
%% PACK DATA FOR UDP OUTPUT (filelogger continuous)
%SF needs to check this for completeness for DM task
taskOutput.continuous = packFileLoggerFormatAndData('continuous', ...
    TASK_NAME, VERSION_ID, ...
    'clock', clock, ...
    'pause', pauseTriggered, ...
    'xpcRequestClock', behaviorRequestClock, ...
    'peripheralTimestamp', peripheralTimestamp, ...
    'state', state, ...
    'inputType', inputType, ...
    'windowsPacketSize', behaviorPacket.windowsPacketSize, ...
    'windowsMousePosition', behaviorPacket.windowsMousePosition, ...
    'windowsTimestamp', behaviorPacket.windowsTimestamp, ...
    'windowsPC1GazePoint', behaviorPacket.windowsPC1GazePoint, ...
    'windowsPC1GazePointValid', behaviorPacket.windowsPC1GazeValid, ...
    'rigidBodyPosXYZ', behaviorPacket.rigidBodyPosXYZ, ...
    'rigidBodyRotXYZ', behaviorPacket.rigidBodyRotXYZ, ...
    'windowsPC1Timestamp', behaviorPacket.windowsPC1Timestamp, ...
    'xpcScreenUpdateClock',vizPacket.xpcScreenUpdateClock,...
    'effectorCursorPos', effectorCursorPos(1:NUM_DIMS), ...
    'currentTarget', single(currentTarget(:,1)), ...
    ...%'currentTargetType', uint16(currentTargetType),...
    'xk', single(taskOutput.xk),...
    'stateTimer', stateTimer, ...
    'holdTimer', holdTimer, ...
    'behaviorPacketSize', behaviorPacket.packetSize, ...
    'xpcTET', single(xpcTET), ...
    'robotTimestamp', behaviorPacket.robotTimestamp, ...
    'gain', decisionParameters.gain, ...  % not locked
    'powerGain', decisionParameters.powerGain, ...
    'powerGainUnityCrossing', decisionParameters.powerGain, ...
    'headCursorPos', headCursorPos(1:NUM_DIMS), ... % always head cursor for DM task
    'xkModBiasEst', single(xkModBiasEst), ... %the bias estimate coming from the bias killer that acts on xkMod (after nonlinear gain)
    'stimCondMatrix', trialConds,...      %entry in stimulus Matrix for trial 
    'activeTargets', activeTargs,...     % DM - tells all targ locs and colors
    'fixDur', fixDur,...
    'targDur', targDur,...
    'successPoints', successPoints... %DM for displaying score  
    );

% Send these all together to conserve bytes, because the names are all
% encoded too.
workspaceAll = [lockedParameters.workspaceX;
    lockedParameters.workspaceY;
    lockedParameters.workspaceZ;
    lockedParameters.workspaceR;
    lockedParameters.workspaceR2];
% added SDS Jan 2016

%% SEND DISCRETE DATA TO FILELOGGER
taskOutput.discrete = packFileLoggerFormatAndData('discrete', ...
    TASK_NAME, VERSION_ID, ...
    'clock', clock,...
    'blockNumber', stateParameters.blockNumber,... 
    'taskType', lockedParameters.taskType, ...
    'targetDiameter', single( targetRadiusTrans*2 ), ...
    'trialDelayLength', trialDelayLength, ...
    'currentTarget', currentTarget,...%I wonder what size this should be... SF
    ...%'speedCode', speedCode,... %for instructed speed experiments
    ...%'holdTime', lockedParameters.holdTime, ...
    'trialNum', trialNum, ...
    'inputType', inputType, ...
    'workspace', workspaceAll, ...
    'outputType', outputType, ...
    'xk2EffectorPosInds', uint8(effectorPosInds(1:NUM_DIMS)), ...  % want to know hor state is being mapped to game horizontal, veritacl, depth, rotate, ...
    'xk2EffectorVelInds', uint8(effectorVelInds(1:NUM_DIMS)), ...
    'selectionRefractoryMS', uint16( lockedParameters.selectionRefractoryMS ), ... % for Gridlike task Added Dec 15 2016 SDS
    'numTargets',  uint16( lockedParameters.numTargets ), ...  % used for RAYS bitrate compute
    'gridSize', lockedParameters.gridSize,... % 1D color matrix edge length in px
    'targetInds', int16(lockedParameters.targetInds(1:4,1:16)), ... % only twoD, 8 targets, to support doing monthly R8/Fitts in PTB from same compiled code.
    'maxStimDur', uint16(lockedParameters.maxStimDur),... % for DM ref
    'maxFixDur', uint16(lockedParameters.maxFixDur),...   % for DM ref
    'maxTargDur', uint16(lockedParameters.maxTargDur),...  % for DM ref
    'taskOrder', uint16(lockedParameters.taskOrder)... % for DM ref. stim first or targets first
    );

%% SEND DATA OUT TO VIZ
taskOutput.screen = packFileLoggerFormatAndData('screen', ...
    TASK_NAME, VERSION_ID, ...
    'clock', clock,...
    'totalTaskTime',totalTaskTime,...
    'blockNumber', stateParameters.blockNumber,...
    'state',state,...
    'cursorPosition',  horzcat(effectorCursorPos(1:NUM_DIMS)', headCursorPos(1:NUM_DIMS)', eyeCursorPos(1:NUM_DIMS)),... % handhold the compiler with dims here
    'cursorColors', lockedParameters.cursorColors,...
    'cursorDiameter', lockedParameters.cursorDiameter,...
    'targetDiameter', single( targetRadiusTrans*2 ),...
    'targetRotDiameter', single( targetRadiusRot*2) ,...
    'targetColor', targetColor, ... %this is 'a', get rid of all 'a' logic
    'inputType', inputType,...
    'drawNumbersOnTargets',lockedParameters.drawNumbersOnTargets,...
    'taskType', lockedParameters.taskType,...
    'recenterDelay', lockedParameters.recenterDelay,...
    'cursorVelocity', cursorVelocity(1:NUM_DIMS), ...
    'outputType', outputType, ...
    'numDisplayDims', lockedParameters.numDisplayDims, ...
    'showXYZaura', lockedParameters.showXYZaura, ... % not logged.
    'displayObject', lockedParameters.displayObject, ... % not logged
    'numTargets',uint8(lockedParameters.numTargets), ... % 
    'targetInds', int16(lockedParameters.targetInds(1:4,1:16)), ... % only twoD, 8 targets, to support doing monthly R8/Fitts in PTB from same compiled code.
    'successPoints', successPoints,... %DM for displaying score
    'activeTargets', activeTargs,...%DM mission critical!! 
    'stimCondMatrix', trialConds,... %entry in stimulus Matrix for trial
    'targetColors', targColors, ....% this is for having 2 targets up
    'makeGrid', makeGridFlag, ... %whether or not to generate a texture
    'gridSize', lockedParameters.gridSize,... % 1D color matrix edge length in px
    'crossSize', lockedParameters.crossSize,... %1D fixation cross width in px
    'taskOrder', lockedParameters.taskOrder... % stim first or targets first
);
% SF found the limits of the size of this guy- keep it below 32 elements
%% SEND DATA OUT TO SOUND
taskOutput.sound = packFileLoggerFormatAndData('screen', ...
    TASK_NAME, VERSION_ID, ...
    'clock', clock,...
    'vizState',state,...
    'lastSoundTime',lastSoundTime,...
    'lastSoundState',lastSoundState...
    );

%% SET SEND FLAGS FOR NETWORK OUTPUTS
if(clock < INIT_TIME)
    taskOutput.discrete.data.send = false;
    taskOutput.continuous.data.send = false;
    taskOutput.screen.data.send = false;
    taskOutput.sound.data.send = false;
    
    if(mod(clock, 10)==0)
        taskOutput.sendFormat = true;
    else
        taskOutput.sendFormat = false;
    end
    stateTimer = uint16(0);
else
    taskOutput.discrete.data.send = writeDiscreteData;
    taskOutput.continuous.data.send = writeContinuousData;
    taskOutput.screen.data.send = true;
    taskOutput.sound.data.send = true;
    taskOutput.sendFormat = false;
    taskOutput.inputType = inputType;
end
taskOutput.wiaCode = wiaCode; %apparently this *has* to stay? why though... SF
taskOutput.speedCode = speedCode;
taskOutput.paused = pauseTriggered;
taskOutput.allowStop = true; % allowStop;
lastState = state;

end %end main 

%% function defs
function vizPacket = parseVizPacket(packetData)

vizPacket.xpcScreenUpdateClock = typecast(packetData(28+[1:4]), 'uint32');

end

function vizPacket = initVizPacket()

vizPacket.xpcScreenUpdateClock = uint32(0);

end

function StimCondMat =  getStimMat(cohD)
% input: vector of desired coherences
% output: matrix of task conditions
% col 1: 2 = L/R, 1 = U/D
% col 2: color of Left/Down targ 2 = red, 3 = green
% col 3: color of right/up targ 2 = red, 3 = green
% col 4: number of red squares (out of 225)
% col 5: which target is correct. 1 = left/down, 2 = right/up
% rng('shuffle');
StimCondMat = makeStimMat(cohD)
% Block randomizer
BlockVTrialOrder = randperm(size(StimCondMat,1));
StimCondMat = StimCondMat(BlockVTrialOrder,:);
end

function stimMat = makeStimMat(cohD)
% make stimCondsMat for desired coherence levels cohD
% the actual coherence will vary to make the num red squares an integer
% num squares total is hardcoded to be 15*15; 
% col 1: 2 = L/R, 1 = U/D
% col 2: color of Left/Down targ 2 = red, 3 = green
% col 3: color of right/up targ 2 = red, 3 = green
% col 4: number of red squares (out of 225)
% col 5: which target is correct. 1 = left/down, 2 = right/up
maxSquares = 15*15; 
numR = zeros(1,length(cohD)); 
cohDcount = 0;
for cidx = cohD 
    cohDcount = cohDcount + 1; 
    numR(cohDcount) = round(((maxSquares*cidx/100)+maxSquares)/2);
end

numR = [numR, (maxSquares - numR)];

col1T = ones(cohDcount*8,1);    % size = numCoh * numAxes * numColors * numTargs
col1T(cohDcount*4+1:end,1) = 2; % target axis index
col23T = [[ones(cohDcount*2,1); ones(cohDcount*2,1)+1]+1, [ones(cohDcount*2,1)+1; ones(cohDcount*2,1)]+1];
col4T = sort(numR, 'descend')'; 
col5T = [ones(cohDcount,1); ones(cohDcount,1)+1; ones(cohDcount,1)+1; ones(cohDcount,1)];
stimMat = [col1T, repmat(col23T, 2,1), repmat(col4T, 4,1), repmat(col5T, 2,1)];  
end

function translateOnTarget = isCursorOnTarget(effectorPos, cursorRadius, targetPosition, targetRadius, TASK_DIMS)
%
% translateOnTarget returns true if at least the translation (dims 1:3)
% are over the target. This can be used to visually depict that
% translation, but not rotation, is correct. - SDS March 2017
useDims = TASK_DIMS;
if sqrt( sum( ((double( effectorPos(1:useDims) ) - double( targetPosition(1:useDims) )).^2 ) ) ) < ...
        double(targetRadius)
    translateOnTarget = true;
else
    translateOnTarget = false;
end
end
